simulink model "Pololu_Motor_Encoder_2018b_Luxi"  (R2018b)
settings: Solver=FixedStepDiscrete  StartTime=0.0  StopTime=10.0  RelTol=1e-3  EnableMultiTasking=on
libraries: c2833xlib x4, c280xlib x4, powerlib_extras x4, fuzblock x1, simulink x1
settings Model: ExtModeTrigDuration=8  Creator=User  LastModifiedBy=User
settings SolverCC: AutoInsertRateTranBlk=on
settings DataIOCC: LimitDataPoints=on  SaveFormat=Array  SaveOutput=off  SaveTime=off
settings OptimizationCC: DefaultUnderspecifiedDataType=single  ExpressionDepthLimit=2147483647  LifeSpan=1  MaxStackSize=512
settings DebuggingCC: UnderspecifiedInitializationDetection=Classic  MergeDetectMultiDrivingBlocksExec=none  SolverPrmCheckMsg=warning  StateNameClashWarn=warning  SFUnexpectedBacktrackingDiag=warning  SFNoUnconditionalDefaultTransitionDiag=warning  SFExecutionAtInitializationDiag=none  UnderSpecifiedDimensionMsg=warning
settings HardwareCC: ProdBitPerChar=16  ProdBitPerInt=16  ProdBitPerPointer=32  ProdBitPerSizeT=32  ProdBitPerPtrDiffT=32  ProdLargestAtomicInteger=Integer  ProdLargestAtomicFloat=None  ProdWordSize=16  ProdLongLongMode=on  ProdHWDeviceType=Texas Instruments->C2000  TargetBitPerChar=16  TargetBitPerInt=16  TargetLargestAtomicInteger=Integer  TargetIntDivRoundTo=Zero  TargetEndianess=LittleEndian  TargetWordSize=16  TargetHWDeviceType=Texas Instruments->C2000  ProdEqTarget=off
settings ModelReferenceCC: PropagateSignalLabelsOutOfModel=off
settings SFSimCC: SimCustomSourceCode="#include \"i2c_reset.c\""  SimCustomHeaderCode="#include \"i2c_reset.h\""  SimUseLocalCustomCode=off  MATLABDynamicMemAlloc=off
settings RTWCC: SystemTargetFile=ert.tlc  HardwareBoard=TI Delfino F2833x  TemplateMakefile=ert_default_tmf  RTWUseLocalCustomCode=off  RTWUseSimCustomCode=on  CustomSourceCode="#include \"i2c_reset.c\""  CustomHeaderCode="#include \"i2c_reset.h\""  Toolchain=Texas Instruments Code Composer Studio (C2000)
settings CodeAppCC: IgnoreCustomStorageClasses=off  CustomSymbolStrType=$N$R$M  StateflowObjectComments=on  InternalIdentifier=Classic
settings ERTTargetCC: CodeReplacementLibrary=TI C28x  MultiwordLength=2048  ParMdlRefBuildCompliant=off  CPPClassGenCompliant=off  ConvertIfToSwitch=off  SuppressUnreachableDefaultCases=off
settings ConfigComp: CovMetricSettings=dw  CovSaveCumulativeToWorkspaceVar=on  CovSaveSingleToWorkspaceVar=on  CovExternalEMLEnable=off

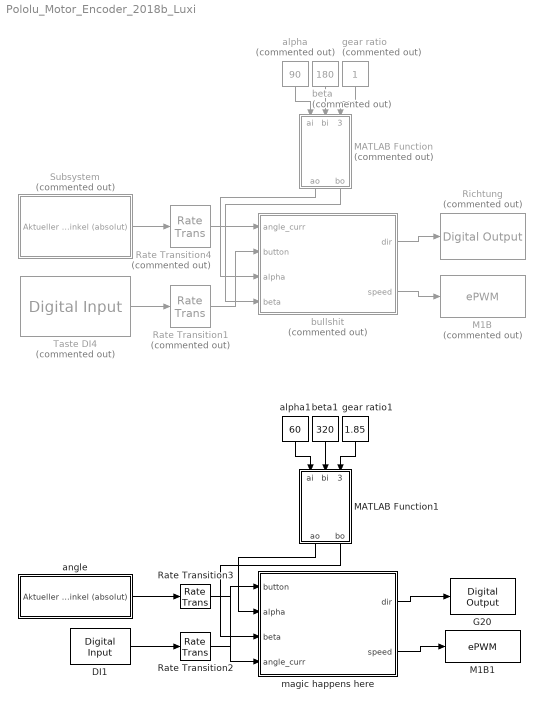
== system Pololu_Motor_Encoder_2018b_Luxi ==
  DI1 : c2833xlib/Digital Input  GPIO_Number=GPIO24~GPIO31  GPIO_Bit0=off  GPIO_Bit1=off  GPIO_Bit2=off  GPIO_Bit3=off  GPIO_Bit4=off  GPIO_Bit5=off  GPIO_Bit6=on  GPIO_Bit7=off  sampleTime=0.1  dataType=auto  GPIO_Bit0_Qualification=Sync to SYSCLKOUT  GPIO_Bit1_Qualification=Sync to SYSCLKOUT  GPIO_Bit2_Qualification=Sync to SYSCLKOUT  GPIO_Bit3_Qualification=Sync to SYSCLKOUT  GPIO_Bit4_Qualification=Sync to SYSCLKOUT  GPIO_Bit5_Qualification=Sync to SYSCLKOUT  GPIO_Bit6_Qualification=Sync to SYSCLKOUT  GPIO_Bit7_Qualification=Sync to SYSCLKOUT  Qualification_Period=-1
      settings: SourceProductBaseCode=TIC2000
  G20 : c2833xlib/Digital Output  GPIO_Number=GPIO16~GPIO23  GPIO_Bit0=off  GPIO_BIT0_Toggle=off  GPIO_Bit1=off  GPIO_BIT1_Toggle=off  GPIO_Bit2=off  GPIO_BIT2_Toggle=off  GPIO_Bit3=off  GPIO_BIT3_Toggle=off  GPIO_Bit4=off  GPIO_BIT4_Toggle=off  GPIO_Bit5=on  GPIO_BIT5_Toggle=off  GPIO_Bit6=off  GPIO_BIT6_Toggle=off  GPIO_Bit7=off  GPIO_BIT7_Toggle=off
      settings: SourceProductBaseCode=TIC2000
  M1B : c280xlib/ePWM  Commented=on  checkMode=off  useModule=ePWM1  periodUnits=Clock cycles  timerSource=Specify via dialog  timerPeriod_clk=64000  timerPeriod_sec=0.0001  tbshadow=Counter equals to zero  countingMode=Up  phaseActiveEnable=Disable  phaseDirection=Count down after sync  phaseActive=0  synchronizationEnable=off  synchronizationOption=Disable  clockPrescale=1  HSclockPrescale=1  ePWMxAStatus=off  CMPAUnits=Clock cycles  CMPASource=Specify via dialog  CMPAValue_per=50  CMPAValue_clk=32000  enCMPAshadow=Counter equals to zero  ePWMxAactionLogic1=Do nothing  ePWMxAactionLogic2=Clear  ePWMxAactionLogic3=Set  ePWMxAactionLogic4=Do nothing  ePWMxAactionLogic5=Do nothing  ePWMxAactionLogic6=Do nothing  ePWMxALoadMode=Load on counter equals to zero (CTR=Zero)  ePWMxACSFenable=off  ePWMxACSFvalue=Forcing disable  ePWMxASFreload=Zero  enHRPWM=off  HRPWM_LoadMode=Counter equals to zero (CTR=ZERO)  HRPWM_CTLMode=Phase control mode  HRPWM_EDGMode=Both edge  enSFO=on  ePWMxBStatus=on  CMPBUnits=Percentages  CMPBSource=Input port  CMPBValue_per=0  CMPBValue_clk=32000  enCMPBshadow=Counter equals to zero  ePWMxBactionLogic1=Do nothing  ePWMxBactionLogic2=Set  ePWMxBactionLogic3=Do nothing  ePWMxBactionLogic4=Do nothing  ePWMxBactionLogic5=Clear  ePWMxBactionLogic6=Do nothing  ePWMxBLoadMode=Load on counter equals to zero (CTR=Zero)  ePWMxBCSFenable=off  ePWMxBCSFvalue=Forcing disable  ePWMxBSFreload=Zero  enableDBePWMxA=off  enableDBePWMxB=off  DBpolarity=Active high (AH)  DBedgeDelay=Positive  DBSource_ePWMxA=ePWMxA  DBSource_ePWMxB=ePWMxA  DBperiodSource=Specify via dialog  REDperiod=0  FEDperiod=0  adcstartModuleA=off  adcrequestEventA=First event  adcstartEventA=Counter equals to zero (CTR=Zero)  adcstartModuleB=off  adcrequestEventB=First event  adcstartEventB=Counter equals to zero (CTR=Zero)  intEn=off  intPrd=First event  intSel=Counter equals to zero (CTR=Zero)  chopperEnable=off  chopperFrequency=1  chopperFirstwidth=1  chopperDuty=12.5%  tripZonesource=Specify via dialog  tzselOSHT1=off  tzselOSHT2=off  tzselOSHT3=off  tzselOSHT4=off  tzselOSHT5=off  tzselOSHT6=off  tzselCBC1=off  tzselCBC2=off  tzselCBC3=off  tzselCBC4=off  tzselCBC5=off  tzselCBC6=off  enTzOstIntr=off  enTzCbcIntr=off  ePWMxAforced=No action  ePWMxBforced=No action  timerPeriod=-1  ePWMxAValue=0  ePWMxBValue=0  tripZoneoption=One-shot trip (OSHT)
      settings: SourceProductBaseCode=TIC2000
  M1B1 : c280xlib/ePWM  checkMode=off  useModule=ePWM2  periodUnits=Clock cycles  timerSource=Specify via dialog  timerPeriod_clk=64000  timerPeriod_sec=0.0001  tbshadow=Counter equals to zero  countingMode=Up  phaseActiveEnable=Disable  phaseDirection=Count down after sync  phaseActive=0  synchronizationEnable=off  synchronizationOption=Disable  clockPrescale=1  HSclockPrescale=1  ePWMxAStatus=off  CMPAUnits=Clock cycles  CMPASource=Specify via dialog  CMPAValue_per=50  CMPAValue_clk=32000  enCMPAshadow=Counter equals to zero  ePWMxAactionLogic1=Do nothing  ePWMxAactionLogic2=Clear  ePWMxAactionLogic3=Set  ePWMxAactionLogic4=Do nothing  ePWMxAactionLogic5=Do nothing  ePWMxAactionLogic6=Do nothing  ePWMxALoadMode=Load on counter equals to zero (CTR=Zero)  ePWMxACSFenable=off  ePWMxACSFvalue=Forcing disable  ePWMxASFreload=Zero  enHRPWM=off  HRPWM_LoadMode=Counter equals to zero (CTR=ZERO)  HRPWM_CTLMode=Phase control mode  HRPWM_EDGMode=Both edge  enSFO=on  ePWMxBStatus=on  CMPBUnits=Percentages  CMPBSource=Input port  CMPBValue_per=0  CMPBValue_clk=32000  enCMPBshadow=Counter equals to zero  ePWMxBactionLogic1=Do nothing  ePWMxBactionLogic2=Set  ePWMxBactionLogic3=Do nothing  ePWMxBactionLogic4=Do nothing  ePWMxBactionLogic5=Clear  ePWMxBactionLogic6=Do nothing  ePWMxBLoadMode=Load on counter equals to zero (CTR=Zero)  ePWMxBCSFenable=off  ePWMxBCSFvalue=Forcing disable  ePWMxBSFreload=Zero  enableDBePWMxA=off  enableDBePWMxB=off  DBpolarity=Active high (AH)  DBedgeDelay=Positive  DBSource_ePWMxA=ePWMxA  DBSource_ePWMxB=ePWMxA  DBperiodSource=Specify via dialog  REDperiod=0  FEDperiod=0  adcstartModuleA=off  adcrequestEventA=First event  adcstartEventA=Counter equals to zero (CTR=Zero)  adcstartModuleB=off  adcrequestEventB=First event  adcstartEventB=Counter equals to zero (CTR=Zero)  intEn=off  intPrd=First event  intSel=Counter equals to zero (CTR=Zero)  chopperEnable=off  chopperFrequency=1  chopperFirstwidth=1  chopperDuty=12.5%  tripZonesource=Specify via dialog  tzselOSHT1=off  tzselOSHT2=off  tzselOSHT3=off  tzselOSHT4=off  tzselOSHT5=off  tzselOSHT6=off  tzselCBC1=off  tzselCBC2=off  tzselCBC3=off  tzselCBC4=off  tzselCBC5=off  tzselCBC6=off  enTzOstIntr=off  enTzCbcIntr=off  ePWMxAforced=No action  ePWMxBforced=No action  timerPeriod=-1  ePWMxAValue=0  ePWMxBValue=0  tripZoneoption=One-shot trip (OSHT)
      settings: SourceProductBaseCode=TIC2000
  MATLAB Function : MATLAB Function  Commented=on  TreatAsAtomicUnit=on
  MATLAB Function1 : MATLAB Function  TreatAsAtomicUnit=on
  Rate Transition1 : RateTransition  Commented=on  OutPortSampleTime=0.01
  Rate Transition2 : RateTransition  OutPortSampleTime=0.0001
  Rate Transition3 : RateTransition  OutPortSampleTime=0.0001
  Rate Transition4 : RateTransition  Commented=on  OutPortSampleTime=0.01
  Richtung : c2833xlib/Digital Output  Commented=on  GPIO_Number=GPIO16~GPIO23  GPIO_Bit0=off  GPIO_BIT0_Toggle=off  GPIO_Bit1=off  GPIO_BIT1_Toggle=off  GPIO_Bit2=off  GPIO_BIT2_Toggle=off  GPIO_Bit3=off  GPIO_BIT3_Toggle=off  GPIO_Bit4=on  GPIO_BIT4_Toggle=off  GPIO_Bit5=off  GPIO_BIT5_Toggle=off  GPIO_Bit6=off  GPIO_BIT6_Toggle=off  GPIO_Bit7=off  GPIO_BIT7_Toggle=off
      settings: SourceProductBaseCode=TIC2000
  Subsystem : Subsystem  Commented=on
  Taste DI4 : c2833xlib/Digital Input  Commented=on  GPIO_Number=GPIO24~GPIO31  GPIO_Bit0=off  GPIO_Bit1=off  GPIO_Bit2=off  GPIO_Bit3=off  GPIO_Bit4=off  GPIO_Bit5=off  GPIO_Bit6=on  GPIO_Bit7=off  sampleTime=0.1  dataType=auto  GPIO_Bit0_Qualification=Sync to SYSCLKOUT  GPIO_Bit1_Qualification=Sync to SYSCLKOUT  GPIO_Bit2_Qualification=Sync to SYSCLKOUT  GPIO_Bit3_Qualification=Sync to SYSCLKOUT  GPIO_Bit4_Qualification=Sync to SYSCLKOUT  GPIO_Bit5_Qualification=Sync to SYSCLKOUT  GPIO_Bit6_Qualification=Sync to SYSCLKOUT  GPIO_Bit7_Qualification=Sync to SYSCLKOUT  Qualification_Period=-1
      settings: SourceProductBaseCode=TIC2000
  alpha : Constant  Commented=on  Value=90
  alpha1 : Constant  Value=60
  angle : Subsystem
  beta : Constant  Commented=on  Value=180
  beta1 : Constant  Value=320
  bullshit : Stateflow chart  Commented=on  TreatAsAtomicUnit=on
  gear ratio : Constant  Commented=on
  gear ratio1 : Constant  Value=1.85
  magic happens here : Stateflow chart  TreatAsAtomicUnit=on
  wires:
  bullshit/2(speed) -> M1B/1
  Taste DI4/1 -> Rate Transition1/1
  Rate Transition4/1 -> bullshit/1(angle_curr)
  Rate Transition1/1 -> bullshit/2(button)
  bullshit/1(dir) -> Richtung/1
  Subsystem/1(Aktueller Winkel (absolut)) -> Rate Transition4/1
  beta/1 -> MATLAB Function/2(bi)
  gear ratio/1 -> MATLAB Function/3(gear_ratio)
  alpha/1 -> MATLAB Function/1(ai)
  MATLAB Function/1(ao) -> bullshit/3(alpha)
  MATLAB Function/2(bo) -> bullshit/4(beta)
  MATLAB Function1/1(ao) -> magic happens here/2(alpha)
  Rate Transition3/1 -> magic happens here/4(angle_curr)
  magic happens here/2(speed) -> M1B1/1
  MATLAB Function1/2(bo) -> magic happens here/3(beta)
  magic happens here/1(dir) -> G20/1
  beta1/1 -> MATLAB Function1/2(bi)
  alpha1/1 -> MATLAB Function1/1(ai)
  gear ratio1/1 -> MATLAB Function1/3(gear_ratio)
  DI1/1 -> Rate Transition2/1
  Rate Transition2/1 -> magic happens here/1(button)
  angle/1(Aktueller Winkel (absolut)) -> Rate Transition3/1

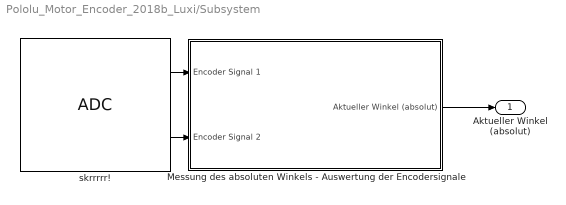
== system Pololu_Motor_Encoder_2018b_Luxi/Subsystem ==
  Messung des absoluten Winkels - Auswertung der Encodersignale : Subsystem
  skrrrrr! : c280xlib/ADC  useModule=A  useMode=Sequential  sourceSOC=Software  sourceSOC1=Software  sourceSOC2=ePWMxB  xint2_ADCSOC=31  Ts=0.00002  dType=double  postInterrupt=off  numConversionsSingle=2  numConversionsDouble=1  conv0=ADCINA0  conv1=ADCINA1  conv2=ADCINA2  conv3=ADCINA3  conv4=ADCINA4  conv5=ADCINA5  conv6=ADCINA6  conv7=ADCINA7  conv8=ADCINB0  conv9=ADCINB1  conv10=ADCINB2  conv11=ADCINB3  conv12=ADCINB4  conv13=ADCINB5  conv14=ADCINB6  conv15=ADCINB7  convAB0=ADCINA0 and ADCINB0  convAB1=ADCINA1 and ADCINB1  convAB2=ADCINA2 and ADCINB2  convAB3=ADCINA3 and ADCINB3  convAB4=ADCINA4 and ADCINB4  convAB5=ADCINA5 and ADCINB5  convAB6=ADCINA6 and ADCINB6  convAB7=ADCINA7 and ADCINB7  convA0=ADCINA0  convA1=ADCINA1  convA2=ADCINA5  convA3=ADCINA3  convA4=ADCINA5  convA5=ADCINA5  convA6=ADCINA6  convA7=ADCINA7  convB0=ADCINB0  convB1=ADCINB1  convB2=ADCINB2  convB3=ADCINB3  convB4=ADCINB4  convB5=ADCINB5  convB6=ADCINB6  convB7=ADCINB7  c28xmultiPort=on  endma=off  chdma=1
      settings: SourceProductBaseCode=TIC2000
  Aktueller Winkel (absolut) : Outport  VectorParamsAs1DForOutWhenUnconnected=on
  wires:
  skrrrrr!/2 -> Messung des absoluten Winkels - Auswertung der Encodersignale/2(Encoder Signal 2)
  skrrrrr!/1 -> Messung des absoluten Winkels - Auswertung der Encodersignale/1(Encoder Signal 1)
  Messung des absoluten Winkels - Auswertung der Encodersignale/1(Aktueller Winkel (absolut)) -> Aktueller Winkel (absolut)/1

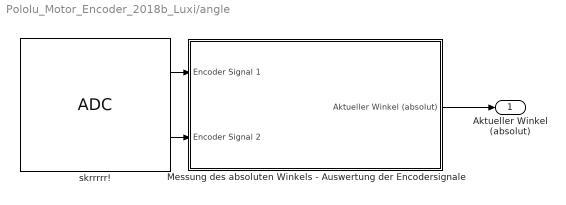
== system Pololu_Motor_Encoder_2018b_Luxi/angle ==
  Messung des absoluten Winkels - Auswertung der Encodersignale : Subsystem
  skrrrrr! : c280xlib/ADC  useModule=A  useMode=Sequential  sourceSOC=Software  sourceSOC1=Software  sourceSOC2=ePWMxB  xint2_ADCSOC=31  Ts=0.00002  dType=double  postInterrupt=off  numConversionsSingle=2  numConversionsDouble=1  conv0=ADCINA0  conv1=ADCINA1  conv2=ADCINA2  conv3=ADCINA3  conv4=ADCINA4  conv5=ADCINA5  conv6=ADCINA6  conv7=ADCINA7  conv8=ADCINB0  conv9=ADCINB1  conv10=ADCINB2  conv11=ADCINB3  conv12=ADCINB4  conv13=ADCINB5  conv14=ADCINB6  conv15=ADCINB7  convAB0=ADCINA0 and ADCINB0  convAB1=ADCINA1 and ADCINB1  convAB2=ADCINA2 and ADCINB2  convAB3=ADCINA3 and ADCINB3  convAB4=ADCINA4 and ADCINB4  convAB5=ADCINA5 and ADCINB5  convAB6=ADCINA6 and ADCINB6  convAB7=ADCINA7 and ADCINB7  convA0=ADCINA0  convA1=ADCINA1  convA2=ADCINA5  convA3=ADCINA3  convA4=ADCINA5  convA5=ADCINA5  convA6=ADCINA6  convA7=ADCINA7  convB0=ADCINB0  convB1=ADCINB1  convB2=ADCINB2  convB3=ADCINB3  convB4=ADCINB4  convB5=ADCINB5  convB6=ADCINB6  convB7=ADCINB7  c28xmultiPort=on  endma=off  chdma=1
      settings: SourceProductBaseCode=TIC2000
  Aktueller Winkel (absolut) : Outport  VectorParamsAs1DForOutWhenUnconnected=on
  wires:
  skrrrrr!/2 -> Messung des absoluten Winkels - Auswertung der Encodersignale/2(Encoder Signal 2)
  skrrrrr!/1 -> Messung des absoluten Winkels - Auswertung der Encodersignale/1(Encoder Signal 1)
  Messung des absoluten Winkels - Auswertung der Encodersignale/1(Aktueller Winkel (absolut)) -> Aktueller Winkel (absolut)/1

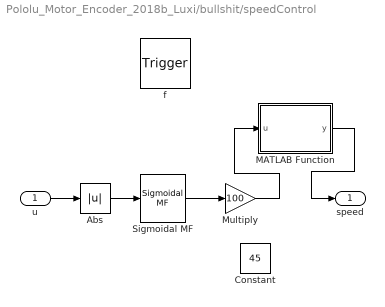
== system Pololu_Motor_Encoder_2018b_Luxi/bullshit/speedControl ==
  u : Inport  OutDataTypeStr=double  PortDimensions=1
  f : TriggerPort  TriggerType=function-call  VariantControl=(inherit)
      settings: CopyFcn=Stateflow.SLINSF.SimulinkMan.removeBlockPreDeleteFcn  PreDeleteFcn=Stateflow.SLINSF.SimulinkMan.unsafePredeleteFcn
  Abs : Abs
  Constant : Constant  Value=45
  MATLAB Function : MATLAB Function  TreatAsAtomicUnit=on
  Multiply : Gain  Gain=100
  Sigmoidal MF : fuzblock/Membership  Functions/Sigmoidal MF  a=0.015  c=60
      settings: SourceProductBaseCode=FL
  speed : Outport  VectorParamsAs1DForOutWhenUnconnected=on
  wires:
  Sigmoidal MF/1 -> Multiply/1
  u/1 -> Abs/1
  Abs/1 -> Sigmoidal MF/1
  Multiply/1 -> MATLAB Function/1(u)
  MATLAB Function/1(y) -> speed/1

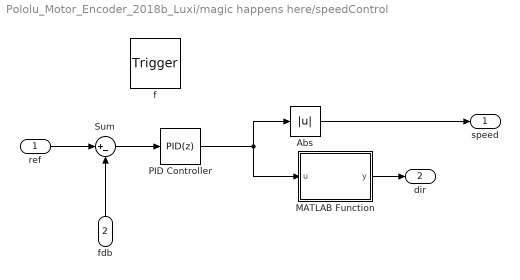
== system Pololu_Motor_Encoder_2018b_Luxi/magic happens here/speedControl ==
  ref : Inport  OutDataTypeStr=double  PortDimensions=1
  fdb : Inport  Port=2  OutDataTypeStr=double  PortDimensions=1
  f : TriggerPort  TriggerType=function-call  VariantControl=(inherit)
      settings: CopyFcn=Stateflow.SLINSF.SimulinkMan.removeBlockPreDeleteFcn  PreDeleteFcn=Stateflow.SLINSF.SimulinkMan.unsafePredeleteFcn
  Abs : Abs
  MATLAB Function : MATLAB Function  TreatAsAtomicUnit=on
  PID Controller : simulink/Continuous/PID Controller  Controller=PID  Form=Parallel  TimeDomain=Discrete-time  SampleTime=-1  IntegratorMethod=Forward Euler  FilterMethod=Forward Euler  ControllerParametersSource=internal  P=4  I=4  D=2  UseFilter=on  N=2000  TunerSelectOption=Transfer Function Based (PID Tuner App)  InitialConditionSource=internal  InitialConditionForIntegrator=0  InitialConditionForFilter=0  DifferentiatorICPrevScaledInput=0  ExternalReset=none  TrackingMode=off  Kt=1  LimitOutput=on  UpperSaturationLimit=100  LowerSaturationLimit=-100  LinearizeAsGain=on  AntiWindupMode=clamping  Kb=5  POutMin=[]  POutMax=[]  IOutMin=[]  IOutMax=[]  DOutMin=[]  DOutMax=[]  NOutMin=[]  NOutMax=[]  SumOutMin=[]  SumOutMax=[]  SaturationOutMin=[]  SaturationOutMax=[]  PParamMin=[]  PParamMax=[]  IParamMin=[]  IParamMax=[]  DParamMin=[]  DParamMax=[]  NParamMin=[]  NParamMax=[]  KbParamMin=[]  KbParamMax=[]  KtParamMin=[]  KtParamMax=[]  KbOutMin=[]  KbOutMax=[]  KtOutMin=[]  KtOutMax=[]  IntegratorOutMin=[]  IntegratorOutMax=[]  FilterOutMin=[]  FilterOutMax=[]  SumI1OutMin=[]  SumI1OutMax=[]  SumI2OutMin=[]  SumI2OutMax=[]  SumI3OutMin=[]  SumI3OutMax=[]  SumI4OutMin=[]  SumI4OutMax=[]  SumDOutMin=[]  SumDOutMax=[]  DifferentiatorOutMin=[]  DifferentiatorOutMax=[]  FilterDiffOutCoefMin=[]  FilterDiffOutCoefMax=[]  ReciprocalOutMin=[]  ReciprocalOutMax=[]  SumDenOutMin=[]  SumDenOutMax=[]  SumNumOutMin=[]  SumNumOutMax=[]  DivideOutMin=[]  DivideOutMax=[]  IntegratorContinuousStateAttributes=''  IntegratorStateMustResolveToSignalObject=off  IntegratorRTWStateStorageClass=Auto  FilterContinuousStateAttributes=''  FilterStateMustResolveToSignalObject=off  FilterRTWStateStorageClass=Auto  ParallelPVariant=InternalParameters  IdealPVariant=Disabled  IVariant=InternalParameters  DVariant=InternalParameters  IntegratorVariant=Discrete  SatVariant=Enabled  AWVariant=DiscClampingParallel  PCopyVariant=Disabled  TRVariant=Disabled  FdbkBlocksVariant=Forward  IdealPFdbkVariant=Disabled  SatFdbkVariant=Disabled  DerivativeFilterVariant=ForwardEulerFilter  NVariant=InternalParameters  NCopyVariant=Disabled  FilterICVariant=InternalICsFilter  IntegratorICVariant=InternalICs  ExternalResetVariant=Disabled  TRSumVariant=Passthrough  SumFdbkVariant=Disabled  SumVariant=Sum_PID
  Sum : Sum  Inputs=|+-
  speed : Outport  VectorParamsAs1DForOutWhenUnconnected=on
  dir : Outport  Port=2  VectorParamsAs1DForOutWhenUnconnected=on
  wires:
  MATLAB Function/1(y) -> dir/1
  fdb/1 -> Sum/2
  ref/1 -> Sum/1
  Sum/1 -> PID Controller/1
  PID Controller/1 -> MATLAB Function/1(u), Abs/1
  Abs/1 -> speed/1

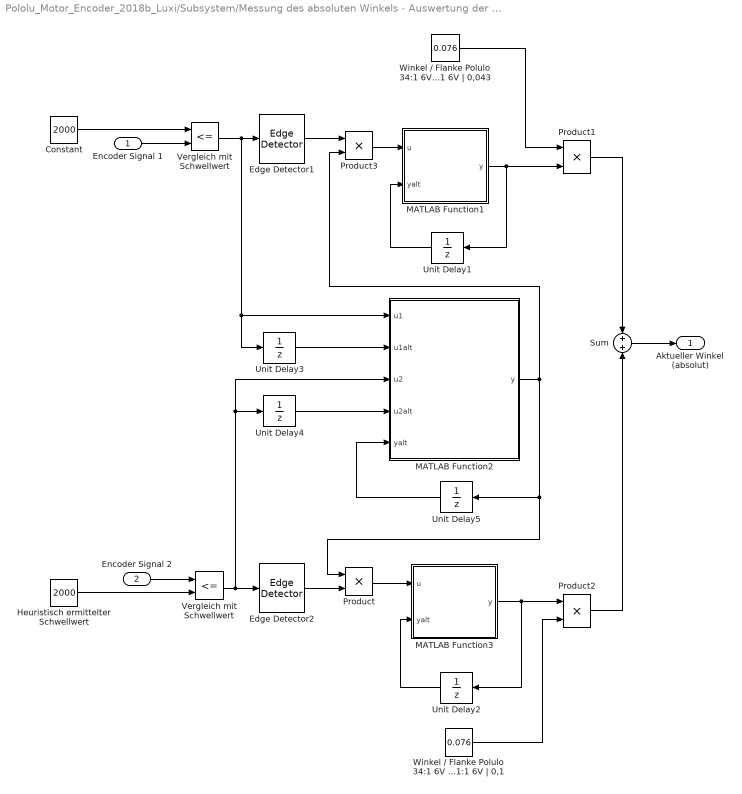
== system Pololu_Motor_Encoder_2018b_Luxi/Subsystem/Messung des absoluten Winkels - Auswertung der Encodersignale ==
  Encoder Signal 1 : Inport
  Encoder Signal 2 : Inport  Port=2
  Constant : Constant  Value=2000
  Edge Detector1 : powerlib_extras/Control  Blocks/Edge Detector  model=Either  ic=0
      settings: SourceProductBaseCode=PS
  Edge Detector2 : powerlib_extras/Control  Blocks/Edge Detector  model=Either  ic=0
      settings: SourceProductBaseCode=PS
  Heuristisch ermittelter Schwellwert : Constant  Value=2000
  MATLAB Function1 : MATLAB Function  TreatAsAtomicUnit=on
  MATLAB Function2 : MATLAB Function  TreatAsAtomicUnit=on
  MATLAB Function3 : MATLAB Function  TreatAsAtomicUnit=on
  Product{,1..3} (4 alike) : Product  RndMeth=Zero
  Sum : Sum  Inputs=+|+
  Unit Delay{1..5} (5 alike) : UnitDelay  SampleTime=-1
  Vergleich mit Schwellwert : RelationalOperator  Operator=<=  OutDataTypeStr=boolean  RndMeth=Nearest
  Vergleich mit Schwellwert : RelationalOperator  Operator=<=  OutDataTypeStr=boolean  RndMeth=Nearest
  Winkel / Flanke Polulo 34:1 6V | 0,22 Polulo 74:1 6V | 0,1 Polulo 98:1 6V | 0,076 Polulo 171:1 6V | 0,043 : Constant  Value=0.076
  Winkel / Flanke Polulo 34:1 6V | 0,22 Polulo 74:1 6V | 0,1 Polulo 98:1 6V | 0,076 Polulo 171:1 6V | 0,1 : Constant  Value=0.076
  Aktueller Winkel (absolut) : Outport
  wires:
  Vergleich mit Schwellwert/1 -> Unit Delay4/1, MATLAB Function2/3(u2), Edge Detector2/1
  Sum/1 -> Aktueller Winkel (absolut)/1
  Vergleich mit Schwellwert/1 -> Edge Detector1/1, Unit Delay3/1, MATLAB Function2/1(u1)
  Heuristisch ermittelter Schwellwert/1 -> Vergleich mit Schwellwert/2
  Unit Delay2/1 -> MATLAB Function3/2(yalt)
  Encoder Signal 1/1 -> Vergleich mit Schwellwert/2
  MATLAB Function3/1(y) -> Unit Delay2/1, Product2/1
  Product1/1 -> Sum/1
  Constant/1 -> Vergleich mit Schwellwert/1
  Encoder Signal 2/1 -> Vergleich mit Schwellwert/1
  Product2/1 -> Sum/2
  Unit Delay1/1 -> MATLAB Function1/2(yalt)
  MATLAB Function1/1(y) -> Product1/2, Unit Delay1/1
  Winkel / Flanke Polulo 34:1 6V | 0,22 Polulo 74:1 6V | 0,1 Polulo 98:1 6V | 0,076 Polulo 171:1 6V | 0,043/1 -> Product1/1
  Product3/1 -> MATLAB Function1/1(u)
  Product/1 -> MATLAB Function3/1(u)
  Edge Detector1/1 -> Product3/1
  Unit Delay3/1 -> MATLAB Function2/2(u1alt)
  Unit Delay4/1 -> MATLAB Function2/4(u2alt)
  Edge Detector2/1 -> Product/2
  MATLAB Function2/1(y) -> Product3/2, Product/1, Unit Delay5/1
  Winkel / Flanke Polulo 34:1 6V | 0,22 Polulo 74:1 6V | 0,1 Polulo 98:1 6V | 0,076 Polulo 171:1 6V | 0,1/1 -> Product2/2
  Unit Delay5/1 -> MATLAB Function2/5(yalt)

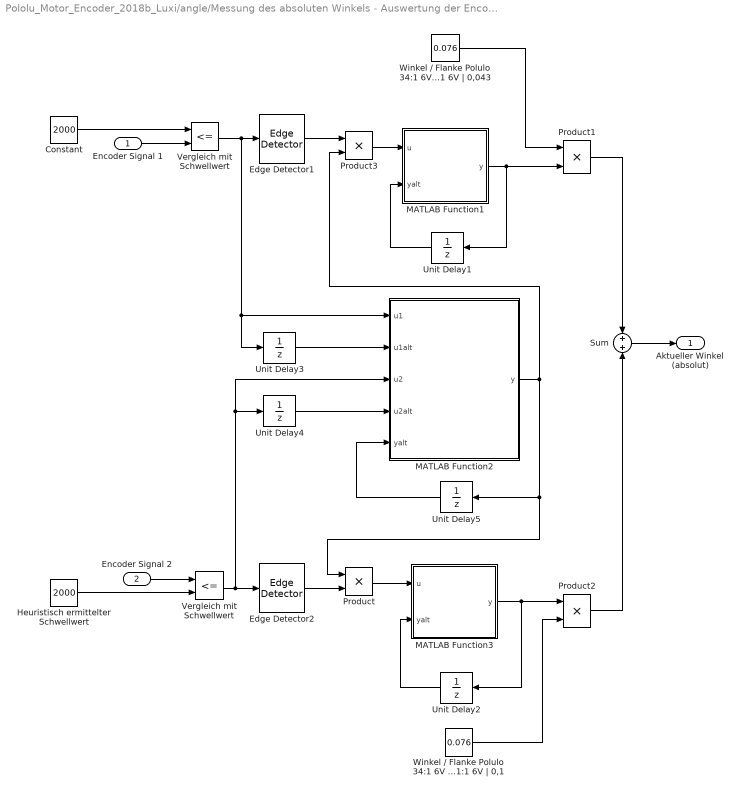
== system Pololu_Motor_Encoder_2018b_Luxi/angle/Messung des absoluten Winkels - Auswertung der Encodersignale ==
  Encoder Signal 1 : Inport
  Encoder Signal 2 : Inport  Port=2
  Constant : Constant  Value=2000
  Edge Detector1 : powerlib_extras/Control  Blocks/Edge Detector  model=Either  ic=0
      settings: SourceProductBaseCode=PS
  Edge Detector2 : powerlib_extras/Control  Blocks/Edge Detector  model=Either  ic=0
      settings: SourceProductBaseCode=PS
  Heuristisch ermittelter Schwellwert : Constant  Value=2000
  MATLAB Function1 : MATLAB Function  TreatAsAtomicUnit=on
  MATLAB Function2 : MATLAB Function  TreatAsAtomicUnit=on
  MATLAB Function3 : MATLAB Function  TreatAsAtomicUnit=on
  Product{,1..3} (4 alike) : Product  RndMeth=Zero
  Sum : Sum  Inputs=+|+
  Unit Delay{1..5} (5 alike) : UnitDelay  SampleTime=-1
  Vergleich mit Schwellwert : RelationalOperator  Operator=<=  OutDataTypeStr=boolean  RndMeth=Nearest
  Vergleich mit Schwellwert : RelationalOperator  Operator=<=  OutDataTypeStr=boolean  RndMeth=Nearest
  Winkel / Flanke Polulo 34:1 6V | 0,22 Polulo 74:1 6V | 0,1 Polulo 98:1 6V | 0,076 Polulo 171:1 6V | 0,043 : Constant  Value=0.076
  Winkel / Flanke Polulo 34:1 6V | 0,22 Polulo 74:1 6V | 0,1 Polulo 98:1 6V | 0,076 Polulo 171:1 6V | 0,1 : Constant  Value=0.076
  Aktueller Winkel (absolut) : Outport
  wires:
  Vergleich mit Schwellwert/1 -> Unit Delay4/1, MATLAB Function2/3(u2), Edge Detector2/1
  Sum/1 -> Aktueller Winkel (absolut)/1
  Vergleich mit Schwellwert/1 -> Edge Detector1/1, Unit Delay3/1, MATLAB Function2/1(u1)
  Heuristisch ermittelter Schwellwert/1 -> Vergleich mit Schwellwert/2
  Unit Delay2/1 -> MATLAB Function3/2(yalt)
  Encoder Signal 1/1 -> Vergleich mit Schwellwert/2
  MATLAB Function3/1(y) -> Unit Delay2/1, Product2/1
  Product1/1 -> Sum/1
  Constant/1 -> Vergleich mit Schwellwert/1
  Encoder Signal 2/1 -> Vergleich mit Schwellwert/1
  Product2/1 -> Sum/2
  Unit Delay1/1 -> MATLAB Function1/2(yalt)
  MATLAB Function1/1(y) -> Product1/2, Unit Delay1/1
  Winkel / Flanke Polulo 34:1 6V | 0,22 Polulo 74:1 6V | 0,1 Polulo 98:1 6V | 0,076 Polulo 171:1 6V | 0,043/1 -> Product1/1
  Product3/1 -> MATLAB Function1/1(u)
  Product/1 -> MATLAB Function3/1(u)
  Edge Detector1/1 -> Product3/1
  Unit Delay3/1 -> MATLAB Function2/2(u1alt)
  Unit Delay4/1 -> MATLAB Function2/4(u2alt)
  Edge Detector2/1 -> Product/2
  MATLAB Function2/1(y) -> Product3/2, Product/1, Unit Delay5/1
  Winkel / Flanke Polulo 34:1 6V | 0,22 Polulo 74:1 6V | 0,1 Polulo 98:1 6V | 0,076 Polulo 171:1 6V | 0,1/1 -> Product2/2
  Unit Delay5/1 -> MATLAB Function2/5(yalt)

== matlab function Pololu_Motor_Encoder_2018b_Luxi/bullshit/speedControl/MATLAB Function ==
  data: u input; y output
function y = limiter45(u)
if u >45
    y=45;
else
    y=u;
end

== matlab function Pololu_Motor_Encoder_2018b_Luxi/MATLAB Function ==
  data: ai input; ao output; bi input; gear_ratio input; bo output
function [ao,bo] = fcn(ai,bi,gear_ratio)
ao=(1/gear_ratio)*ai;
bo=(1/gear_ratio)*bi;

== stateflow chart Pololu_Motor_Encoder_2018b_Luxi/bullshit ==
  state bla
    angle_init=angle_curr;
  state On1
    dir=1;
    speed=speedControl(absDiff(angle_init,angle_curr)-alpha);
  state stage_alpha
    speed=0;
    dir=1;
  state init
  state stage1
    speed=speedControl(absDiff(angle_init,angle_curr)-beta);
  state speed = speedControl(u) [function]
  state stage2
    speed=speedControl(absDiff(angle_init,angle_curr)-alpha);
  state stage_beta
    speed=0;
    dir=0;
  bla -> On1 : [after(2,sec)]
  stage_alpha -> stage1 : after(5,sec)
  On1 -> stage_alpha : [absDiff(angle_init,angle_curr)>=alpha]
  init -> bla : [button == 1]
  (default) -> init
  stage1 -> stage_beta : [absDiff(angle_init,angle_curr)>=beta]
  stage2 -> stage_alpha : [absDiff(angle_init,angle_curr)<=alpha]
  stage_beta -> stage2 : after(5,sec)
  data: speed function_output; u function_input double size=1; u function_input; v function_input; ad function_output; angle_curr input double; dir output; speed output; button input boolean; alpha input; beta input; angle_init local
  function ad=absDiff(u,v):
    | function ad=absDiff(u,v)
    |  ad = abs(abs(u)-abs(v));

== matlab function Pololu_Motor_Encoder_2018b_Luxi/MATLAB Function1 ==
  data: ai input; ao output; bi input; gear_ratio input; bo output
function [ao,bo] = fcn(ai,bi,gear_ratio)
ao=(gear_ratio)*ai;
bo=(gear_ratio)*bi;

== matlab function Pololu_Motor_Encoder_2018b_Luxi/angle/Messung des absoluten Winkels - Auswertung der Encodersignale/MATLAB Function1 ==
  data: u input; y output; yalt input
function y = fcn(u, yalt)

y = yalt + u;

== matlab function Pololu_Motor_Encoder_2018b_Luxi/angle/Messung des absoluten Winkels - Auswertung der Encodersignale/MATLAB Function2 ==
  data: u1 input; u1alt input; u2 input; u2alt input; y output; yalt input double
function y = fcn(u1, u1alt, u2, u2alt, yalt)

y = 1;

if u1alt == 0 && u2alt == 0 && u1 == 0 && u2 == 0
    y = yalt;
end

if u1alt == 0 && u2alt == 0 && u1 == 0 && u2 == 1
    y = 1;
end

if u1alt == 0 && u2alt == 0 && u1 == 1 && u2 == 0
    y = -1;
end

% if u1alt == 0 && u2alt == 0 && u1 == 1 && u2 == 1
%     y = yalt;   % nicht möglich
% end

if u1alt == 0 && u2alt == 1 && u1 == 0 && u2 == 0
    y = -1;
end

if u1alt == 0 && u2alt == 1 && u1 == 0 && u2 == 1
    y = yalt;
end

% if u1alt == 0 && u2alt == 1 && u1 == 1 && u2 == 0
%     y = yalt;   % nicht möglich
% end

if u1alt == 0 && u2alt == 1 && u1 == 1 && u2 == 1
    y = 1;
end

if u1alt == 1 && u2alt == 0 && u1 == 0 && u2 == 0
    y = 1;
end

% if u1alt == 1 && u2alt == 0 && u1 == 0 && u2 == 1
%     y = yalt;   % nicht möglich
% end

if u1alt == 1 && u2alt == 0 && u1 == 1 && u2 == 0
    y = yalt;
end

if u1alt == 1 && u2alt == 0 && u1 == 1 && u2 == 1
    y = -1;
end

% if u1alt == 1 && u2alt == 1 && u1 == 0 && u2 == 0
%     y = yalt;   % nicht möglich
% end

if u1alt == 1 && u2alt == 1 && u1 == 0 && u2 == 1
    y = -1;
end

if u1alt == 1 && u2alt == 1 && u1 == 1 && u2 == 0
    y = 1;
end

if u1alt == 1 && u2alt == 1 && u1 == 1 && u2 == 1
    y = yalt;
end
end

== matlab function Pololu_Motor_Encoder_2018b_Luxi/angle/Messung des absoluten Winkels - Auswertung der Encodersignale/MATLAB Function3 ==
  data: u input; y output; yalt input
function y = fcn(u, yalt)

y = yalt + u;

== matlab function Pololu_Motor_Encoder_2018b_Luxi/Subsystem/Messung des absoluten Winkels - Auswertung der Encodersignale/MATLAB Function1 ==
  data: u input; y output; yalt input
function y = fcn(u, yalt)

y = yalt + u;

== stateflow chart Pololu_Motor_Encoder_2018b_Luxi/magic happens here ==
  state init2
    angle_init=angle_curr;
  state init
  state goAlpha
    [speed,dir]=speedControl(angle_init + alpha,angle_curr);
  state weird
    speed=0;
  state weird1
    speed=0;
  state [speed,dir] = speedControl(ref,fdb) [function]
  state goBeta
    [speed,dir]=speedControl(angle_init + beta,angle_curr);
  note: angle_current=absDiff(angle_init,angle_curr,alpha);
  init -> init2 : [button == 1]
  (default) -> init
  init2 -> goAlpha : [after(5,sec)]
  weird -> goAlpha : [after(5,sec)]
  goAlpha -> weird1 : [absDiff(angle_init,angle_curr,alpha)<=3]
  goBeta -> weird : [absDiff(angle_init,angle_curr,beta)<=3]
  weird1 -> goBeta : [after(5,sec)]
  data: speed function_output; ref function_input double size=1; fdb function_input double size=1; dir function_output; u function_input; v function_input; ad function_output; z function_input; dir output; speed output; button input boolean; alpha input; beta input; angle_curr input double; angle_init local
  function ad=absDiff(u,v,z):
    | function ad=absDiff(u,v,z)
    |  tmp = abs(abs(u)-abs(v));
    |  ad = abs(tmp - abs(z));

== matlab function Pololu_Motor_Encoder_2018b_Luxi/magic happens here/speedControl/MATLAB Function ==
  data: u input; y output
function y = oneOrZero(u)
if u >= 0
    y = 1;
else
    y = 0;
end

== matlab function Pololu_Motor_Encoder_2018b_Luxi/Subsystem/Messung des absoluten Winkels - Auswertung der Encodersignale/MATLAB Function2 ==
  data: u1 input; u1alt input; u2 input; u2alt input; y output; yalt input double
function y = fcn(u1, u1alt, u2, u2alt, yalt)

y = 1;

if u1alt == 0 && u2alt == 0 && u1 == 0 && u2 == 0
    y = yalt;
end

if u1alt == 0 && u2alt == 0 && u1 == 0 && u2 == 1
    y = 1;
end

if u1alt == 0 && u2alt == 0 && u1 == 1 && u2 == 0
    y = -1;
end

% if u1alt == 0 && u2alt == 0 && u1 == 1 && u2 == 1
%     y = yalt;   % nicht möglich
% end

if u1alt == 0 && u2alt == 1 && u1 == 0 && u2 == 0
    y = -1;
end

if u1alt == 0 && u2alt == 1 && u1 == 0 && u2 == 1
    y = yalt;
end

% if u1alt == 0 && u2alt == 1 && u1 == 1 && u2 == 0
%     y = yalt;   % nicht möglich
% end

if u1alt == 0 && u2alt == 1 && u1 == 1 && u2 == 1
    y = 1;
end

if u1alt == 1 && u2alt == 0 && u1 == 0 && u2 == 0
    y = 1;
end

% if u1alt == 1 && u2alt == 0 && u1 == 0 && u2 == 1
%     y = yalt;   % nicht möglich
% end

if u1alt == 1 && u2alt == 0 && u1 == 1 && u2 == 0
    y = yalt;
end

if u1alt == 1 && u2alt == 0 && u1 == 1 && u2 == 1
    y = -1;
end

% if u1alt == 1 && u2alt == 1 && u1 == 0 && u2 == 0
%     y = yalt;   % nicht möglich
% end

if u1alt == 1 && u2alt == 1 && u1 == 0 && u2 == 1
    y = -1;
end

if u1alt == 1 && u2alt == 1 && u1 == 1 && u2 == 0
    y = 1;
end

if u1alt == 1 && u2alt == 1 && u1 == 1 && u2 == 1
    y = yalt;
end
end

== matlab function Pololu_Motor_Encoder_2018b_Luxi/Subsystem/Messung des absoluten Winkels - Auswertung der Encodersignale/MATLAB Function3 ==
  data: u input; y output; yalt input
function y = fcn(u, yalt)

y = yalt + u;
